simulink model "step4"  (R2026a)
settings: Solver=VariableStepAuto  StopTime=30
undefined symbols (not defined in the file or in its folder): A, Cd, m, rho, theta
libraries: simulink x4
settings Model: Creator=manoj  LastModifiedBy=manoj

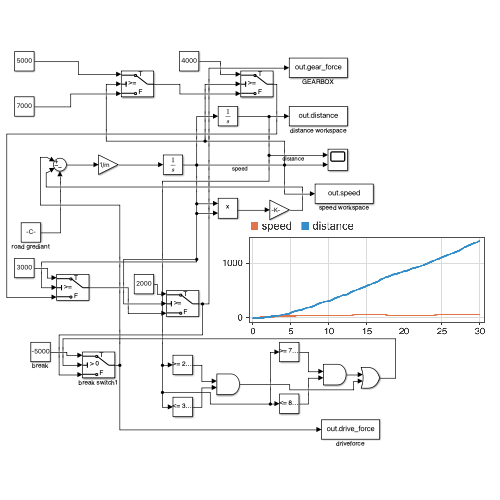
[thumbnail: Simulink's stored preview of the top-level diagram]
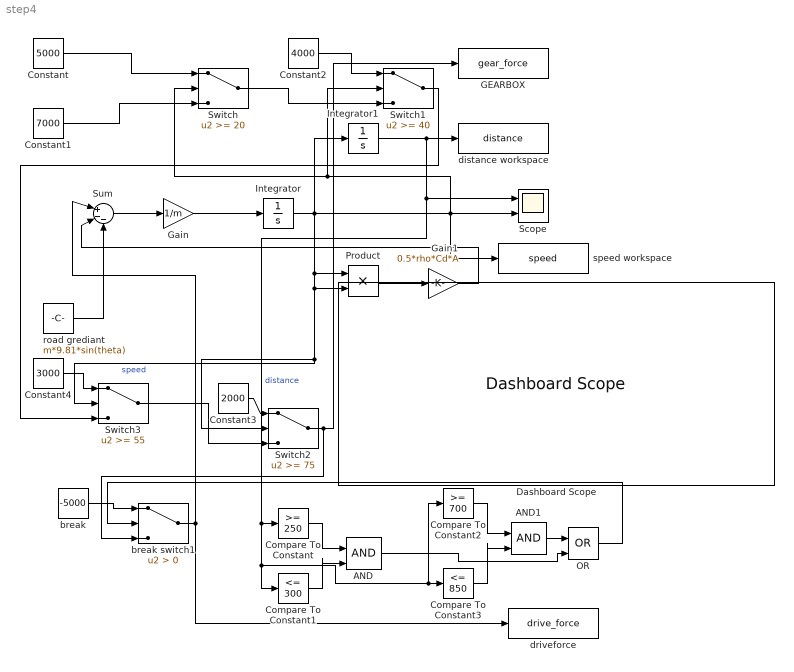
== system step4 ==
  AND : Logic  IconShape=distinctive  AllPortsSameDT=off  OutDataTypeStr=boolean
  AND1 : Logic  IconShape=distinctive  AllPortsSameDT=off  OutDataTypeStr=boolean
  Compare To Constant : simulink/Logic and Bit Operations/Compare To Constant  relop=>=  const=250  OutDataTypeStr=boolean
  Compare To Constant1 : simulink/Logic and Bit Operations/Compare To Constant  relop=<=  const=300  OutDataTypeStr=boolean
  Compare To Constant2 : simulink/Logic and Bit Operations/Compare To Constant  relop=>=  const=700  OutDataTypeStr=boolean
  Compare To Constant3 : simulink/Logic and Bit Operations/Compare To Constant  relop=<=  const=850  OutDataTypeStr=boolean
  Constant : Constant  Value=5000
  Constant1 : Constant  Value=7000
  Constant2 : Constant  Value=4000
  Constant3 : Constant  Value=2000
  Constant4 : Constant  Value=3000
  Dashboard Scope : DashboardScope  FontColor=[0.0, 0.0, 0.0]
  GEARBOX : ToWorkspace  VariableName=gear_force  SaveFormat=Structure With Time  SampleTime=-1
  Gain : Gain  Gain=1/m
  Gain1 : Gain  Gain=0.5*rho*Cd*A
  Integrator : Integrator
  Integrator1 : Integrator
  OR : Logic  Operator=OR  IconShape=distinctive  AllPortsSameDT=off  OutDataTypeStr=boolean
  Product : Product
  Scope : Scope  NumInputPorts=2
      settings: ActiveDisplayYMinimum=-1  ActiveDisplayYMaximum=1
  Sum : Sum  Inputs=|+--
  Switch : Switch  Threshold=20  SaturateOnIntegerOverflow=off  InputSameDT=off
  Switch1 : Switch  Threshold=40  SaturateOnIntegerOverflow=off  InputSameDT=off
  Switch2 : Switch  Threshold=75  ZeroCross=off  SaturateOnIntegerOverflow=off  InputSameDT=off
  Switch3 : Switch  Threshold=55  SaturateOnIntegerOverflow=off  InputSameDT=off
  break : Constant  Value=-5000
  break switch1 : Switch  Criteria=u2 > Threshold  SaturateOnIntegerOverflow=off  InputSameDT=off
  distance workspace : ToWorkspace  VariableName=distance  SaveFormat=Structure With Time  SampleTime=-1
  driveforce : ToWorkspace  VariableName=drive_force  SaveFormat=Structure With Time  SampleTime=-1
  road grediant : Constant  Value=m*9.81*sin(theta)
  speed workspace : ToWorkspace  VariableName=speed  SaveFormat=Structure With Time  SampleTime=-1
  wires:
  road grediant/1 -> Sum/3
  Sum/1 -> Gain/1
  Integrator/1 -> Switch3/2, Switch2/2, Product/2, Product/1, Integrator1/1, Switch1/2, Switch/2, Scope/2, speed workspace/1  "speed"
  Gain/1 -> Integrator/1
  Product/1 -> Gain1/1
  Integrator1/1 -> Compare To Constant1/1, Compare To Constant2/1, Compare To Constant3/1, Compare To Constant/1, Scope/1, distance workspace/1  "distance"
  Gain1/1 -> Sum/2
  Constant/1 -> Switch/1
  Constant1/1 -> Switch/3
  Constant2/1 -> Switch1/1
  Switch/1 -> Switch1/3
  Switch1/1 -> Switch3/3
  Switch3/1 -> Switch2/3
  Constant3/1 -> Switch2/1
  Switch2/1 -> break switch1/3, GEARBOX/1
  Constant4/1 -> Switch3/1
  break/1 -> break switch1/1
  break switch1/1 -> driveforce/1, Sum/1
  Compare To Constant/1 -> AND/1
  Compare To Constant1/1 -> AND/2
  Compare To Constant2/1 -> AND1/1
  Compare To Constant3/1 -> AND1/2
  AND1/1 -> OR/1
  AND/1 -> OR/2
  OR/1 -> break switch1/2
